simulink model "SoC_measurement_ETR07"  (R2017b)
settings: Solver=FixedStepAuto  StartTime=0.0  StopTime=10.0  RelTol=1e-3
settings Model: Creator=cspt  LastModifiedBy=cspt
settings RTWCC: SystemTargetFile=irt.tlc  TemplateMakefile=irt_default_tmf  Description=INTECRIO Real-Time Target
settings STFCustomTargetCC: TargetLangStandard=C99 (ISO)  UtilityFuncGeneration=Shared location  SystemTargetFile=irt.tlc
settings GRTTargetCC: UtilityFuncGeneration=Shared location  ParMdlRefBuildCompliant=off  CompOptLevelCompliant=off  ConcurrentExecutionCompliant=off  CombineOutputUpdateFcns=off  MatFileLogging=off  CPPClassGenCompliant=off  GRTInterface=on  UseToolchainInfoCompliant=off  GenerateASAP2=on

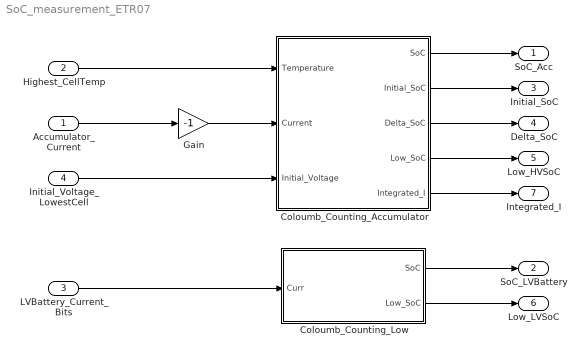
== system SoC_measurement_ETR07 ==
  Accumulator_Current : Inport
  Highest_CellTemp : Inport  Port=2
  LVBattery_Current_Bits : Inport  Port=3
  Initial_Voltage_LowestCell : Inport  Port=4
  Coloumb_Counting_Accumulator : Subsystem
  Coloumb_Counting_Low : Subsystem
  Gain : Gain  Gain=-1
  SoC_Acc : Outport
  SoC_LVBattery : Outport  Port=2
  Initial_SoC : Outport  Port=3
  Delta_SoC : Outport  Port=4
  Low_HVSoC : Outport  Port=5
  Low_LVSoC : Outport  Port=6
  Integrated_I : Outport  Port=7
  wires:
  Coloumb_Counting_Accumulator/1(SoC) -> SoC_Acc/1
  Accumulator_Current/1 -> Gain/1
  Gain/1 -> Coloumb_Counting_Accumulator/2(Current)
  Highest_CellTemp/1 -> Coloumb_Counting_Accumulator/1(Temperature)
  Coloumb_Counting_Low/1(SoC) -> SoC_LVBattery/1
  LVBattery_Current_Bits/1 -> Coloumb_Counting_Low/1(Curr)
  Initial_Voltage_LowestCell/1 -> Coloumb_Counting_Accumulator/3(Initial_Voltage)
  Coloumb_Counting_Accumulator/2(Initial_SoC) -> Initial_SoC/1
  Coloumb_Counting_Accumulator/3(Delta_SoC) -> Delta_SoC/1
  Coloumb_Counting_Accumulator/4(Low_SoC) -> Low_HVSoC/1
  Coloumb_Counting_Low/2(Low_SoC) -> Low_LVSoC/1
  Coloumb_Counting_Accumulator/5(Integrated_I) -> Integrated_I/1

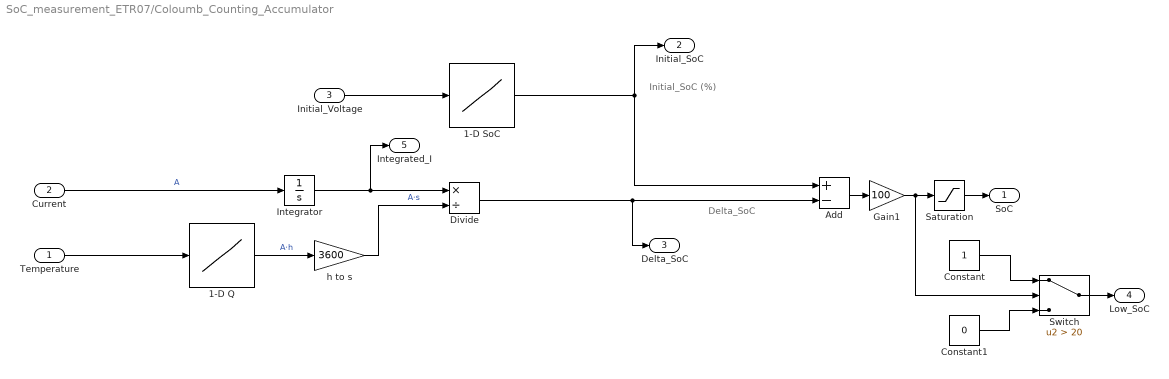
== system SoC_measurement_ETR07/Coloumb_Counting_Accumulator ==
  note: Initial_SoC (%)
  note: Delta_SoC
  Temperature : Inport
  Current : Inport  Port=2
  Initial_Voltage : Inport  Port=3
  1-D Q : Lookup_n-D  NumberOfTableDimensions=1  BreakpointsForDimension1=[5 15 25 35 45 55]  Table="[7.07624408200000\t7.05038665100000\t7.04592614500000\t7.03618918500000\t7.00214276800000\t7.00214276800000]"  InternalRulePriority=Speed  RndMeth=Simplest  InputSameDT=on
  1-D SoC : Lookup_n-D  NumberOfTableDimensions=1  BreakpointsForDimension1="[2.92500000000000\t2.98500000000000\t3.06200000000000\t3.12100000000000\t3.17300000000000\t3.21900000000000\t3.25900000000000\t3.29600000000000\t3.32900000000000\t3.35900000000000\t3.38700000000000\t3.41200000000000\t3.43600000000000\t3.45800000000000\t3.47900000000000\t3.49800000000000\t3.51600000000000\t3.53300000000000\t3.54900000000000\t3.56300000000000\t3.57500000000000\t3.58300000000000\t3.58600000000000\t3.58900000000000\t3.59100000000000\t3.59300000000000\t3.59600000000000\t3.59800000000000\t3.60100000000000\t3.60300000000000\t3.60600000000000\t3.60900000000000\t3.61200000000000\t3.61600000000000\t3.61900000000000\t3.62300000000000\t3.62700000000000\t3.63200000000000\t3.63700000000000\t3.64200000000000\t3.64800000000000\t3.65400000000000\t3.66000000000000\t3.66600000000000\t3.67200000000000\t3.67800000000000\t3.68400000000000\t3.69000000000000\t3.69600000000000\t3.70200000000000\t3.70900000000000\t3.71600000000000\t3.72200000000000\t3.72800000000000\t3.73400000000000\t3.74000000000000\t3.74600000000000\t3.75300000000000\t3.76000000000000\t3.76700000000000\t3.77400000000000\t3.78100000000000\t3.78700000000000\t3.79200000000000\t3.79600000000000\t3.80100000000000\t3.80500000000000\t3.81000000000000\t3.81400000000000\t3.81800000000000\t3.82200000000000\t3.82600000000000\t3.82900000000000\t3.83300000000000\t3.83600000000000\t3.84000000000000\t3.84300000000000\t3.84700000000000\t3.85000000000000\t3.85300000000000\t3.85600000000000\t3.85900000000000\t3.86200000000000\t3.86500000000000\t3.86800000000000\t3.87000000000000\t3.87300000000000\t3.87600000000000\t3.87800000000000\t3.88100000000000\t3.88300000000000\t3.88600000000000\t3.88800000000000\t3.89000000000000\t3.89300000000000\t3.89500000000000\t3.89800000000000\t3.90000000000000\t3.90200000000000\t3.90500000000000\t3.90700000000000\t3.90900000000000\t3.91100000000000\t3.91300000000000\t3.91600000000000\t3.91800000000000\t3.92000000000000\t3.92200000000000\t3.92400000000000\t3.92600000000000\t3.92800000000000\t3.93000000000000\t3.93300000000000\t3.93500000000000\t3.93700000000000\t3.93900000000000\t3.94100000000000\t3.94400000000000\t3.94600000000000\t3.94800000000000\t3.95100000000000\t3.95300000000000\t3.95500000000000\t3.95800000000000\t3.96000000000000\t3.96300000000000\t3.96600000000000\t3.96900000000000\t3.97100000000000\t3.97400000000000\t3.97800000000000\t3.98100000000000\t3.98500000000000\t3.98900000000000\t3.99300000000000\t3.99700000000000\t4.00200000000000\t4.00600000000000\t4.01100000000000\t4.01500000000000\t4.02000000000000\t4.02400000000000\t4.02900000000000\t4.03300000000000\t4.03600000000000\t4.04000000000000\t4.04400000000000\t4.04700000000000\t4.05000000000000\t4.05300000000000\t4.05600000000000\t4.05900000000000\t4.06100000000000\t4.06400000000000\t4.06600000000000\t4.06800000000000\t4.07100000000000\t4.07300000000000\t4.07500000000000\t4.07700000000000\t4.07900000000000\t4.08000000000000\t4.08200000000000\t4.08400000000000\t4.08500000000000\t4.08700000000000\t4.08900000000000\t4.09000000000000\t4.09200000000000\t4.09300000000000\t4.09500000000000\t4.09600000000000\t4.09800000000000\t4.10000000000000\t4.10200000000000\t4.10300000000000\t4.10500000000000\t4.10700000000000\t4.10900000000000\t4.11100000000000\t4.11300000000000\t4.11500000000000\t4.11700000000000\t4.12000000000000\t4.12200000000000\t4.12500000000000\t4.12800000000000\t4.13100000000000\t4.13400000000000\t4.13700000000000\t4.14100000000000\t4.14400000000000\t4.14800000000000\t4.15300000000000\t4.15800000000000\t4.16300000000000\t4.16800000000000\t4.17400000000000\t4.18100000000000\t4.18800000000000\t4.19900000000000]"  Table=[0:0.005:1]  InternalRulePriority=Speed  RndMeth=Simplest  InputSameDT=on
  Add : Sum  Inputs=+-
  Constant : Constant
  Constant1 : Constant  Value=0
  Divide : Product  Inputs=*/
  Gain1 : Gain  Gain=100
  Integrator : Integrator
  Saturation : Saturate  UpperLimit=100  LowerLimit=0
  Switch : Switch  Criteria=u2 > Threshold  Threshold=20
  h to s : Gain  Gain=3600
  SoC : Outport
  Initial_SoC : Outport  Port=2
  Delta_SoC : Outport  Port=3
  Low_SoC : Outport  Port=4
  Integrated_I : Outport  Port=5
  wires:
  Divide/1 -> Delta_SoC/1, Add/2
  Current/1 -> Integrator/1  "A"
  1-D Q/1 -> h to s/1  "A·h"
  Temperature/1 -> 1-D Q/1
  h to s/1 -> Divide/2  "A·s"
  Initial_Voltage/1 -> 1-D SoC/1
  Saturation/1 -> SoC/1
  Integrator/1 -> Integrated_I/1, Divide/1
  Switch/1 -> Low_SoC/1
  Add/1 -> Gain1/1
  Constant1/1 -> Switch/3
  Constant/1 -> Switch/1
  1-D SoC/1 -> Add/1, Initial_SoC/1
  Gain1/1 -> Saturation/1, Switch/2

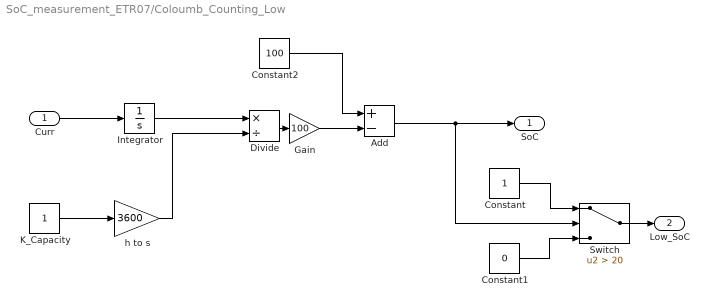
== system SoC_measurement_ETR07/Coloumb_Counting_Low ==
  Curr : Inport
  Add : Sum  Inputs=+-
  Constant : Constant
  Constant1 : Constant  Value=0
  Constant2 : Constant  Value=100
  Divide : Product  Inputs=*/
  Gain : Gain  Gain=100
  Integrator : Integrator
  K_Capacity : Constant
  Switch : Switch  Criteria=u2 > Threshold  Threshold=20
  h to s : Gain  Gain=3600
  SoC : Outport
  Low_SoC : Outport  Port=2
  wires:
  Divide/1 -> Gain/1
  Curr/1 -> Integrator/1
  K_Capacity/1 -> h to s/1
  Integrator/1 -> Divide/1
  h to s/1 -> Divide/2
  Constant/1 -> Switch/1
  Constant1/1 -> Switch/3
  Switch/1 -> Low_SoC/1
  Add/1 -> Switch/2, SoC/1
  Gain/1 -> Add/2
  Constant2/1 -> Add/1
